simulink model "robust_model"  (R2023b)
settings: Solver=VariableStepAuto  StartTime=0.0  StopTime=20  MaxStep=0.01  RelTol=1e-5
values from neighbouring files (symbols this model uses):
  F_alt = 0*M_alt*diag([-0.1, -0.1])    [init_robust_simulink.m]
  Q_M = lftForMInv(M_alt, 0, 0.3)    [init_robust_simulink.m]
undefined symbols (not defined in the file or in its folder): B_alt, E_alt
libraries: cstblocks x12
settings Model: Creator=torb  LastModifiedBy=torb
settings OptimizationCC: DefaultParameterBehavior=Inlined  BufferReuse=off
settings DebuggingCC: InitInArrayFormatMsg=none

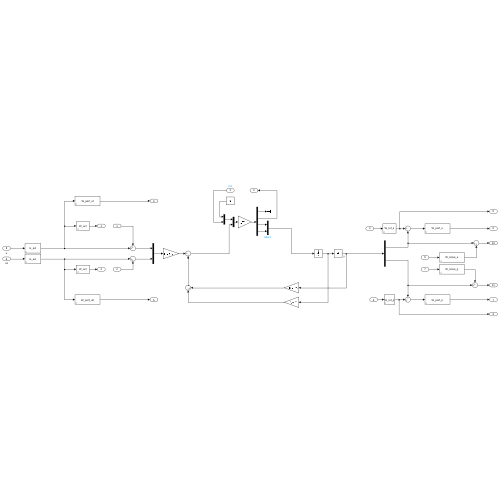
[thumbnail: Simulink's stored preview of the top-level diagram]
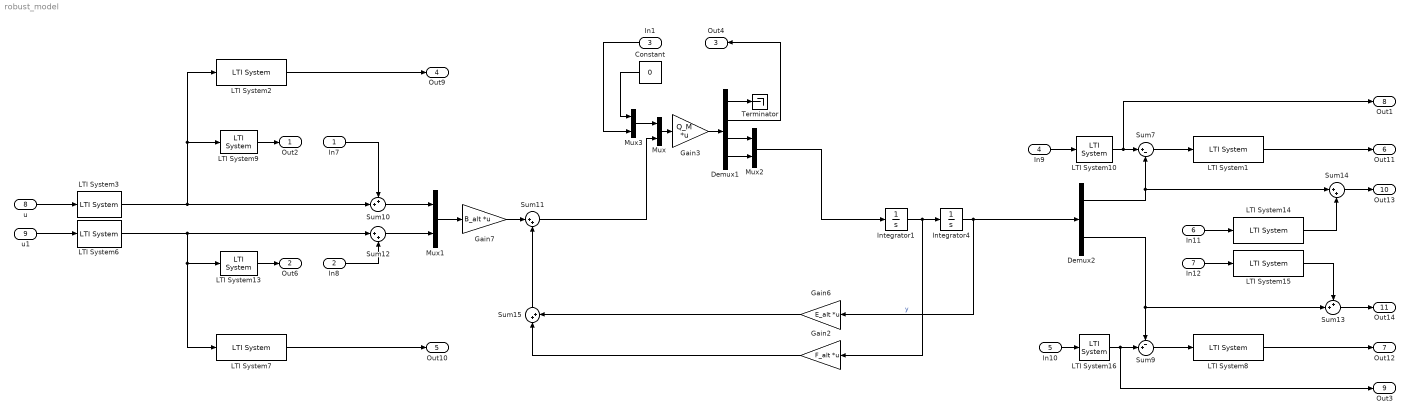
== system robust_model ==
  In7 : Inport
  In8 : Inport  Port=2
  In1 : Inport  Port=3
  In9 : Inport  Port=4
  In10 : Inport  Port=5
  In11 : Inport  Port=6
  In12 : Inport  Port=7
  u : Inport  Port=8
  u1 : Inport  Port=9
  Constant : Constant  Value=0
  Demux1 : Demux
  Demux2 : Demux  Outputs=2
  Gain2 : Gain  Gain=F_alt  Multiplication=Matrix(K*u)
  Gain3 : Gain  Gain=Q_M  Multiplication=Matrix(K*u)
  Gain6 : Gain  Gain=E_alt  Multiplication=Matrix(K*u)
  Gain7 : Gain  Gain=B_alt  Multiplication=Matrix(K*u)
  Integrator1 : Integrator
  Integrator4 : Integrator
  LTI System1 : cstblocks/LTI System  sys=W_perf_e  IC=[]  PadeOrder=0
  LTI System10 : cstblocks/LTI System  sys=W_ref_e  IC=[]  PadeOrder=0
  LTI System13 : cstblocks/LTI System  sys=W_act  IC=[]  PadeOrder=0
  LTI System14 : cstblocks/LTI System  sys=W_noise_e  IC=[]  PadeOrder=0
  LTI System15 : cstblocks/LTI System  sys=W_noise_p  IC=[]  PadeOrder=0
  LTI System16 : cstblocks/LTI System  sys=W_ref_p  IC=[]  PadeOrder=0
  LTI System2 : cstblocks/LTI System  sys=W_perf_uf  IC=[]  PadeOrder=0
  LTI System3 : cstblocks/LTI System  sys=G_act  IC=[]  PadeOrder=0
  LTI System6 : cstblocks/LTI System  sys=G_act  IC=[]  PadeOrder=0
  LTI System7 : cstblocks/LTI System  sys=W_perf_ub  IC=[]  PadeOrder=0
  LTI System8 : cstblocks/LTI System  sys=W_perf_p  IC=[]  PadeOrder=0
  LTI System9 : cstblocks/LTI System  sys=W_act  IC=[]  PadeOrder=0
  Mux{,1..3} (4 alike) : Mux  Inputs=2
  Sum10 : Sum  Inputs=++|
  Sum{11..12,14..15} (4 alike) : Sum  Inputs=|++
  Sum13 : Sum  Inputs=++|
  Sum7 : Sum  Inputs=|+-
  Sum9 : Sum  Inputs=-+|
  Terminator : Terminator
  Out2 : Outport
  Out6 : Outport  Port=2
  Out4 : Outport  Port=3
  Out9 : Outport  Port=4
  Out10 : Outport  Port=5
  Out11 : Outport  Port=6
  Out12 : Outport  Port=7
  Out1 : Outport  Port=8
  Out3 : Outport  Port=9
  Out13 : Outport  Port=10
  Out14 : Outport  Port=11
  wires:
  LTI System3/1 -> Sum10/2, LTI System9/1, LTI System2/1
  LTI System13/1 -> Out6/1
  LTI System9/1 -> Out2/1
  In7/1 -> Sum10/1
  LTI System15/1 -> Sum13/1
  LTI System16/1 -> Sum9/2, Out3/1
  In8/1 -> Sum12/2
  In11/1 -> LTI System14/1
  Demux2/1 -> Sum14/1, Sum7/2
  In10/1 -> LTI System16/1
  LTI System2/1 -> Out9/1
  LTI System7/1 -> Out10/1
  Sum12/1 -> Mux1/2
  Gain7/1 -> Sum11/1
  In12/1 -> LTI System15/1
  LTI System10/1 -> Sum7/1, Out1/1
  LTI System8/1 -> Out12/1
  Demux2/2 -> Sum13/2, Sum9/1
  u1/1 -> LTI System6/1
  u/1 -> LTI System3/1
  Sum10/1 -> Mux1/1
  Sum13/1 -> Out14/1
  Sum15/1 -> Sum11/2
  Mux1/1 -> Gain7/1
  Gain2/1 -> Sum15/1
  Sum9/1 -> LTI System8/1
  LTI System6/1 -> Sum12/1, LTI System13/1, LTI System7/1
  LTI System14/1 -> Sum14/2
  Gain6/1 -> Sum15/2
  Integrator4/1 -> Demux2/1, Gain6/1  "y"
  Sum14/1 -> Out13/1
  Integrator1/1 -> Gain2/1, Integrator4/1
  LTI System1/1 -> Out11/1
  Sum7/1 -> LTI System1/1
  In9/1 -> LTI System10/1
  Demux1/3 -> Mux2/1
  Demux1/4 -> Mux2/2
  Mux3/1 -> Mux/1
  Mux/1 -> Gain3/1
  Gain3/1 -> Demux1/1
  Mux2/1 -> Integrator1/1
  Sum11/1 -> Mux/2
  In1/1 -> Mux3/2
  Demux1/2 -> Out4/1
  Demux1/1 -> Terminator/1
  Constant/1 -> Mux3/1
